simulink model "torque"  (R2016a)
settings: Solver=VariableStepAuto  StartTime=0.0  StopTime=14819  RelTol=1e-3
values from neighbouring files (symbols this model uses):
  freq_range = 1022.16    [torque_converter.m]
  freq_zero = -38.15    [torque_converter.m]
  slope = 15.81    [torque_converter.m]
undefined symbols (not defined in the file or in its folder): parameters
settings Model: Creator=Mark  LastModifiedBy=Mark

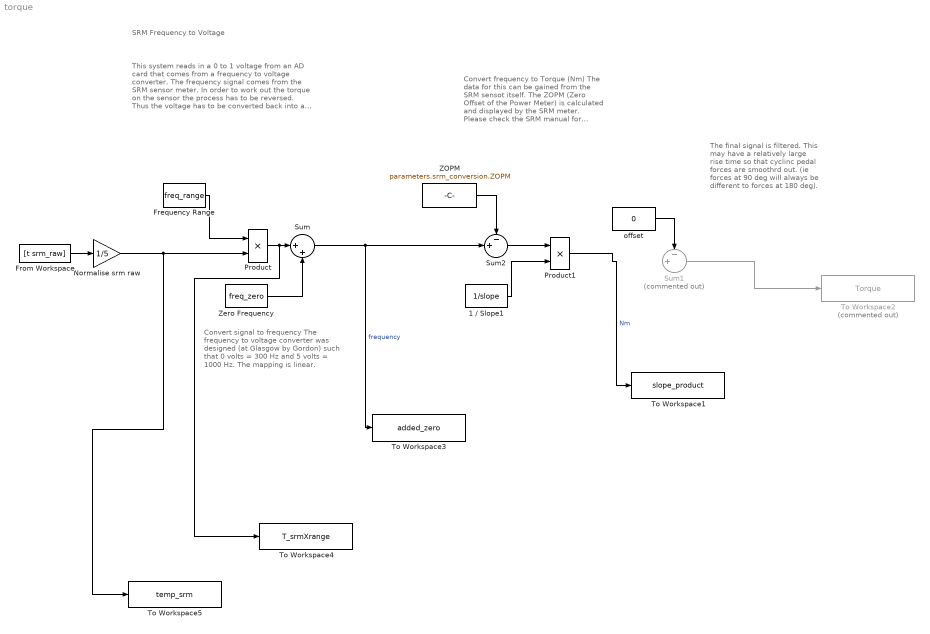
== system torque ==
  note: Convert frequency to Torque (Nm)
      |
      | The data for this can be gained
      | from the SRM sensot itself. The
      | ZOPM (Zero Offset of the Power
      | Meter) is calculated and displayed
      | by the SRM meter.  Please check
      | the SRM manual for details. The
      | 'Slope' value can be read from the
      | back of the SRM sensor.
  note: SRM Frequency to Voltage
  note: This system reads in a 0 to 1 voltage
      | from an AD card that comes from a
      | frequency to voltage converter.  The
      | frequency signal comes from the SRM
      | sensor meter.  In order to work out the
      | torque on the sensor the process has
      | to be reversed.  Thus the voltage has
      | to be converted back into a frequency
      | and then back into a torque.
  note: Convert signal to frequency
      |
      | The frequency to voltage converter
      | was designed (at Glasgow by
      | Gordon) such that 0 volts = 300 Hz
      | and 5 volts = 1000 Hz.  The
      | mapping is linear.
  note: The final signal is filtered.
      | This may have a relatively
      | large rise time so that
      | cyclinc pedal forces are
      | smoothrd out. (ie forces at
      | 90 deg will always be
      | different to forces at 180
      | deg).
  1 / Slope1 : Constant  Value=1/slope
  Frequency Range : Constant  Value=freq_range
  From Workspace : FromWorkspace  VariableName=[t srm_raw]  SampleTime=0
  Normalise srm raw : Gain  Gain=1/5  SaturateOnIntegerOverflow=on  OutDataTypeStr=Inherit: Same as input  ParamDataTypeStr=Inherit: Same as input
  Product : Product  SaturateOnIntegerOverflow=on  InputSameDT=on  OutDataTypeStr=Inherit: Same as first input
  Product1 : Product  SaturateOnIntegerOverflow=on  InputSameDT=on  OutDataTypeStr=Inherit: Same as first input
  Sum : Sum  Inputs=|++  SaturateOnIntegerOverflow=on  InputSameDT=on  OutDataTypeStr=Inherit: Same as first input
  Sum1 : Sum  Commented=on  Inputs=-+|  SaturateOnIntegerOverflow=on  InputSameDT=on  OutDataTypeStr=Inherit: Same as first input
  Sum2 : Sum  Inputs=-+|  SaturateOnIntegerOverflow=on  InputSameDT=on  OutDataTypeStr=Inherit: Same as first input
  To Workspace1 : ToWorkspace  VariableName=slope_product  SampleTime=parameters.sample_time
  To Workspace2 : ToWorkspace  Commented=on  VariableName=Torque  SampleTime=parameters.sample_time
  To Workspace3 : ToWorkspace  VariableName=added_zero  SampleTime=parameters.sample_time
  To Workspace4 : ToWorkspace  VariableName=T_srmXrange  SampleTime=parameters.sample_time
  To Workspace5 : ToWorkspace  VariableName=temp_srm  SampleTime=parameters.sample_time
  ZOPM : Constant  Value=parameters.srm_conversion.ZOPM
  Zero Frequency : Constant  Value=freq_zero
  offset : Constant  Value=0
  wires:
  Zero Frequency/1 -> Sum/2
  1 / Slope1/1 -> Product1/2
  ZOPM/1 -> Sum2/1
  Frequency Range/1 -> Product/1
  Sum/1 -> To Workspace3/1, Sum2/2  "frequency"
  Product/1 -> To Workspace4/1, Sum/1
  Sum2/1 -> Product1/1
  Product1/1 -> To Workspace1/1  "Nm"
  Sum1/1 -> To Workspace2/1
  offset/1 -> Sum1/1
  From Workspace/1 -> Normalise srm raw/1
  Normalise srm raw/1 -> To Workspace5/1, Product/2
